simulink model "Final_Model"  (R2021b)
settings: Solver=FixedStepAuto  StartTime=0.0  StopTime=230  FixedStep=0.1  RelTol=1e-3
values from neighbouring files (symbols this model uses):
  a = 0.6215    [Constant_Params.m]    (also in HIghSpeedMatlabFile.m = 0.65; RearSteer_SideSlipMin.m = 0.7)
  b = 0.5085    [Constant_Params.m]    (also in HIghSpeedMatlabFile.m = 0.6; RearSteer_SideSlipMin.m = 0.62)
  Cf = 33000    [Constant_Params.m]    (also in HIghSpeedMatlabFile.m = 89.892; RearSteer_SideSlipMin.m = 89.892)
  Cr = 34000    [Constant_Params.m]    (also in HIghSpeedMatlabFile.m = 89.892; RearSteer_SideSlipMin.m = 89.892)
  m = 230    [Constant_Params.m]    (also in HIghSpeedMatlabFile.m; RearSteer_SideSlipMin.m)
settings Model: Creator=Hp  LastModifiedBy=Hp

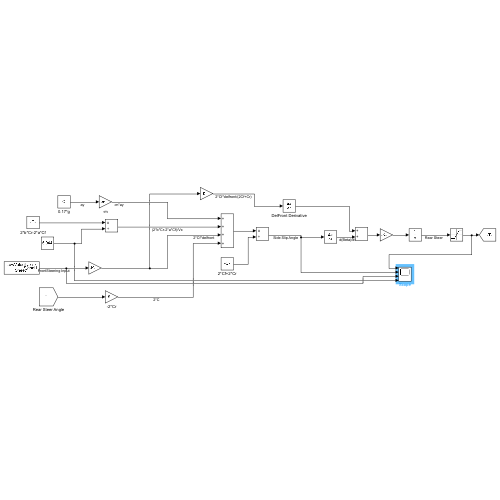
[thumbnail: Simulink's stored preview of the top-level diagram]
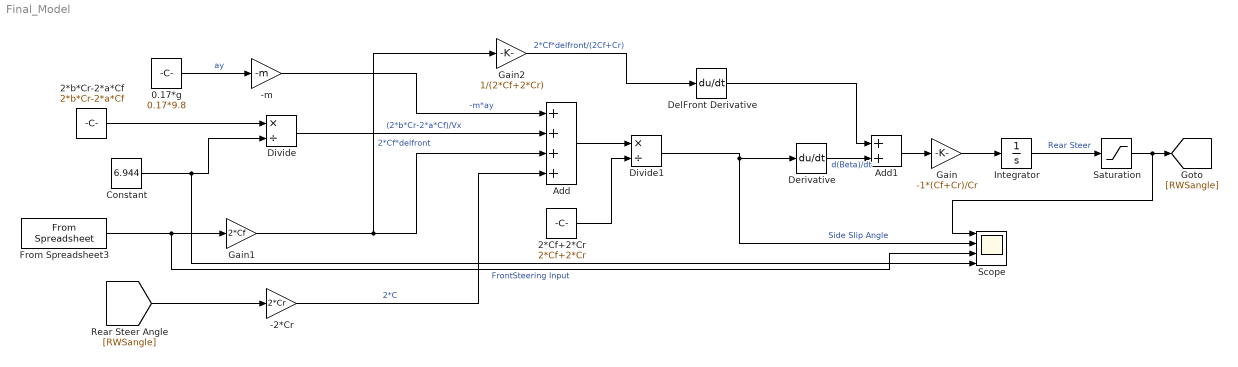
== system Final_Model ==
  -2*Cr : Gain  Gain=2*Cr
  -m : Gain  Gain=-m
  0.17*g : Constant  Value=0.17*9.8
  2*Cf+2*Cr : Constant  Value=2*Cf+2*Cr
  2*b*Cr-2*a*Cf : Constant  Value=2*b*Cr-2*a*Cf
  Add : Sum  Inputs=++++
  Add1 : Sum
  Constant : Constant  Value=6.944
  DelFront Derivative : Derivative
  Derivative : Derivative
  Divide : Product  Inputs=*/
  Divide1 : Product  Inputs=*/
  From Spreadsheet3 : FromSpreadsheet  FileName=LowVelocity.xlsx
  Gain : Gain  Gain=-1*(Cf+Cr)/Cr
  Gain1 : Gain  Gain=2*Cf
  Gain2 : Gain  Gain=1/(2*Cf+2*Cr)
  Integrator : Integrator
  Saturation : Saturate  UpperLimit=6  LowerLimit=-6  LinearizeAsGain=off  ZeroCross=off  RndMeth=Ceiling
  Scope : Scope  NumInputPorts=4
  wires:
  0.17*g/1 -> -m/1  "ay"
  -m/1 -> Add/1  "-m*ay"
  Constant/1 -> Scope/4, Divide/2
  2*b*Cr-2*a*Cf/1 -> Divide/1
  [RWSangle] -> -2*Cr/1
  -2*Cr/1 -> Add/4  "2*C"
  Divide/1 -> Add/2  "(2*b*Cr-2*a*Cf)/Vx"
  Gain1/1 -> Gain2/1, Add/3  "2*Cf*delfront"
  Add/1 -> Divide1/1
  2*Cf+2*Cr/1 -> Divide1/2
  Divide1/1 -> Derivative/1, Scope/2  "Side Slip Angle"
  Gain/1 -> Integrator/1
  Integrator/1 -> Saturation/1  "Rear Steer"
  Saturation/1 -> Scope/1, [RWSangle]
  From Spreadsheet3/1 -> Scope/3, Gain1/1  "FrontSteering Input"
  Gain2/1 -> DelFront Derivative/1  "2*Cf*delfront/(2Cf+Cr)"
  DelFront Derivative/1 -> Add1/1
  Add1/1 -> Gain/1
  Derivative/1 -> Add1/2  "d(Beta)/dt"
